simulink model "IEEE9_case"  (R2024b)
settings: Solver=FixedStepAuto  StartTime=0  StopTime=5  FixedStep=1e-7  RelTol=1e-3
values from neighbouring files (symbols this model uses):
  SG_D_1_D = 0.01056    [IEEE9_case_parameters.m]    (also in case1_parameters.m; case2_parameters.m; case3_parameters.m; case4_parameters.m)
  SG_D_1_EnableSaturation = 0    [IEEE9_case_parameters.m]    (also in case1_parameters.m; case2_parameters.m; case3_parameters.m; case4_parameters.m)
  SG_D_1_f0 = 60    [IEEE9_case_parameters.m]    (also in case1_parameters.m; case2_parameters.m; case3_parameters.m; case4_parameters.m)
  SG_D_1_H = 7.5    [IEEE9_case_parameters.m]    (also in case1_parameters.m; case2_parameters.m; case3_parameters.m; case4_parameters.m)
  SG_D_1_K_A = 20    [IEEE9_case_parameters.m]    (also in case1_parameters.m; case2_parameters.m; case3_parameters.m; case4_parameters.m)
  SG_D_1_K_E = 1.000000e+1    (= 10)    [IEEE9_case_parameters.m]    (also in case1_parameters.m; case2_parameters.m; case3_parameters.m; case4_parameters.m)
  SG_D_1_K_F = 2.363    [IEEE9_case_parameters.m]    (also in case1_parameters.m; case2_parameters.m; case3_parameters.m; case4_parameters.m)
  SG_D_1_K_s = 0.5    [IEEE9_case_parameters.m]    (also in case1_parameters.m = 5; case2_parameters.m = 5; case3_parameters.m = 5; case4_parameters.m = 5)
  SG_D_1_R_a = 0.001088    [IEEE9_case_parameters.m]    (also in case1_parameters.m; case2_parameters.m; case3_parameters.m; case4_parameters.m)
  SG_D_1_S_A = 1    [IEEE9_case_parameters.m]    (also in case1_parameters.m; case2_parameters.m; case3_parameters.m; case4_parameters.m)
  SG_D_1_S_B = 0.103    [IEEE9_case_parameters.m]    (also in case1_parameters.m; case2_parameters.m; case3_parameters.m; case4_parameters.m)
  SG_D_1_S_N = 10.659857    [IEEE9_case_parameters.m]    (also in case1_parameters.m; case2_parameters.m; case3_parameters.m; case4_parameters.m)
  SG_D_1_SpeedPara = 200    [IEEE9_case_parameters.m]    (also in case1_parameters.m; case2_parameters.m; case3_parameters.m; case4_parameters.m)
  SG_D_1_T_0 = 0.720173    [IEEE9_case_parameters.m]    (also in case1_parameters.m = 0.755522; case2_parameters.m = 0.808931; case3_parameters.m = 0.869402; case4_parameters.m = 0.729316)
  SG_D_1_T_1 = 0.3    [IEEE9_case_parameters.m]    (also in case1_parameters.m; case2_parameters.m; case3_parameters.m; case4_parameters.m)
  SG_D_1_T_2 = 0.05    [IEEE9_case_parameters.m]    (also in case1_parameters.m; case2_parameters.m; case3_parameters.m; case4_parameters.m)
  SG_D_1_T_3 = 0.02    [IEEE9_case_parameters.m]    (also in case1_parameters.m; case2_parameters.m; case3_parameters.m; case4_parameters.m)
  SG_D_1_T_4 = 0.005    [IEEE9_case_parameters.m]    (also in case1_parameters.m; case2_parameters.m; case3_parameters.m; case4_parameters.m)
  SG_D_1_T_A = 0.02    [IEEE9_case_parameters.m]    (also in case1_parameters.m; case2_parameters.m; case3_parameters.m; case4_parameters.m)
  SG_D_1_T_dd = 8.000000e+0    (= 8)    [IEEE9_case_parameters.m]    (also in case1_parameters.m; case2_parameters.m; case3_parameters.m; case4_parameters.m)
  SG_D_1_T_ddd = 0.04    [IEEE9_case_parameters.m]    (also in case1_parameters.m; case2_parameters.m; case3_parameters.m; case4_parameters.m)
  SG_D_1_T_E = 0.314    [IEEE9_case_parameters.m]    (also in case1_parameters.m; case2_parameters.m; case3_parameters.m; case4_parameters.m)
  SG_D_1_T_F = 0.35    [IEEE9_case_parameters.m]    (also in case1_parameters.m; case2_parameters.m; case3_parameters.m; case4_parameters.m)
  SG_D_1_T_qd = 0.8    [IEEE9_case_parameters.m]    (also in case1_parameters.m; case2_parameters.m; case3_parameters.m; case4_parameters.m)
  SG_D_1_T_qdd = 0.02    [IEEE9_case_parameters.m]    (also in case1_parameters.m; case2_parameters.m; case3_parameters.m; case4_parameters.m)
  SG_D_1_T_speed = 0.1    [IEEE9_case_parameters.m]    (also in case1_parameters.m = 200; case2_parameters.m = 200; case3_parameters.m = 200; case4_parameters.m = 200)
  SG_D_1_T_w = 0.5    [IEEE9_case_parameters.m]    (also in case1_parameters.m; case2_parameters.m; case3_parameters.m; case4_parameters.m)
  SG_D_1_V_ref = 1.990276    [IEEE9_case_parameters.m]    (also in case1_parameters.m = 2.042296; case2_parameters.m = 2.051388; case3_parameters.m = 2.089584; case4_parameters.m = 2.01845)
  SG_D_1_w_ref = 376.991118    [IEEE9_case_parameters.m]    (also in case1_parameters.m; case2_parameters.m; case3_parameters.m; case4_parameters.m)
  SG_D_1_wb = 6.000000e+1    (= 60)    [IEEE9_case_parameters.m]    (also in case1_parameters.m; case2_parameters.m; case3_parameters.m; case4_parameters.m)
  SG_D_1_x_d = 1.9    [IEEE9_case_parameters.m]    (also in case1_parameters.m; case2_parameters.m; case3_parameters.m; case4_parameters.m)
  SG_D_1_x_dd = 0.302    [IEEE9_case_parameters.m]    (also in case1_parameters.m; case2_parameters.m; case3_parameters.m; case4_parameters.m)
  SG_D_1_x_ddd = 0.204    [IEEE9_case_parameters.m]    (also in case1_parameters.m; case2_parameters.m; case3_parameters.m; case4_parameters.m)
  SG_D_1_x_l = 0.05    [IEEE9_case_parameters.m]    (also in case1_parameters.m; case2_parameters.m; case3_parameters.m; case4_parameters.m)
  SG_D_1_x_q = 1.3    [IEEE9_case_parameters.m]    (also in case1_parameters.m; case2_parameters.m; case3_parameters.m; case4_parameters.m)
  SG_D_1_x_qd = 0.5    [IEEE9_case_parameters.m]    (also in case1_parameters.m; case2_parameters.m; case3_parameters.m; case4_parameters.m)
  SG_D_1_x_qdd = 0.3    [IEEE9_case_parameters.m]    (also in case1_parameters.m; case2_parameters.m; case3_parameters.m; case4_parameters.m)
  SG_D_2_D = 0.02    [IEEE9_case_parameters.m]    (also in case1_parameters.m; case2_parameters.m; case3_parameters.m; case4_parameters.m)
  SG_D_2_EnableSaturation = 0    [IEEE9_case_parameters.m]    (also in case1_parameters.m; case2_parameters.m; case3_parameters.m; case4_parameters.m)
  SG_D_2_f0 = 60    [IEEE9_case_parameters.m]    (also in case1_parameters.m; case2_parameters.m; case3_parameters.m; case4_parameters.m)
  SG_D_2_H = 8.000000e+0    (= 8)    [IEEE9_case_parameters.m]    (also in case1_parameters.m; case2_parameters.m; case3_parameters.m; case4_parameters.m)
  SG_D_2_K_A = 20    [IEEE9_case_parameters.m]    (also in case1_parameters.m; case2_parameters.m; case3_parameters.m; case4_parameters.m)
  SG_D_2_K_E = 1.000000e+1    (= 10)    [IEEE9_case_parameters.m]    (also in case1_parameters.m; case2_parameters.m; case3_parameters.m; case4_parameters.m)
  SG_D_2_K_F = 2.363    [IEEE9_case_parameters.m]    (also in case1_parameters.m; case2_parameters.m; case3_parameters.m; case4_parameters.m)
  SG_D_2_K_s = 0.5    [IEEE9_case_parameters.m]    (also in case1_parameters.m = 4; case2_parameters.m = 4; case3_parameters.m = 4; case4_parameters.m = 4)
  SG_D_2_R_a = 0.001088    [IEEE9_case_parameters.m]    (also in case1_parameters.m; case2_parameters.m; case3_parameters.m; case4_parameters.m)
  SG_D_2_S_A = 1    [IEEE9_case_parameters.m]    (also in case1_parameters.m; case2_parameters.m; case3_parameters.m; case4_parameters.m)
  SG_D_2_S_B = 0.103    [IEEE9_case_parameters.m]    (also in case1_parameters.m; case2_parameters.m; case3_parameters.m; case4_parameters.m)
  SG_D_2_S_N = 10.659857    [IEEE9_case_parameters.m]    (also in case1_parameters.m; case2_parameters.m; case3_parameters.m; case4_parameters.m)
  SG_D_2_SpeedPara = 200    [IEEE9_case_parameters.m]    (also in case1_parameters.m; case2_parameters.m; case3_parameters.m; case4_parameters.m)
  SG_D_2_T_0 = 1.632913    [IEEE9_case_parameters.m]    (also in case1_parameters.m = 1.632925; case2_parameters.m = 1.632915; case3_parameters.m = 1.632914; case4_parameters.m = 1.632927)
  SG_D_2_T_1 = 0.2    [IEEE9_case_parameters.m]    (also in case1_parameters.m; case2_parameters.m; case3_parameters.m; case4_parameters.m)
  SG_D_2_T_2 = 0.05    [IEEE9_case_parameters.m]    (also in case1_parameters.m; case2_parameters.m; case3_parameters.m; case4_parameters.m)
  SG_D_2_T_3 = 0.02    [IEEE9_case_parameters.m]    (also in case1_parameters.m; case2_parameters.m; case3_parameters.m; case4_parameters.m)
  SG_D_2_T_4 = 0.005    [IEEE9_case_parameters.m]    (also in case1_parameters.m; case2_parameters.m; case3_parameters.m; case4_parameters.m)
  SG_D_2_T_A = 0.02    [IEEE9_case_parameters.m]    (also in case1_parameters.m; case2_parameters.m; case3_parameters.m; case4_parameters.m)
  SG_D_2_T_dd = 7.9    [IEEE9_case_parameters.m]    (also in case1_parameters.m; case2_parameters.m; case3_parameters.m; case4_parameters.m)
  SG_D_2_T_ddd = 0.04    [IEEE9_case_parameters.m]    (also in case1_parameters.m; case2_parameters.m; case3_parameters.m; case4_parameters.m)
  SG_D_2_T_E = 0.314    [IEEE9_case_parameters.m]    (also in case1_parameters.m; case2_parameters.m; case3_parameters.m; case4_parameters.m)
  SG_D_2_T_F = 0.35    [IEEE9_case_parameters.m]    (also in case1_parameters.m; case2_parameters.m; case3_parameters.m; case4_parameters.m)
  SG_D_2_T_qd = 0.8    [IEEE9_case_parameters.m]    (also in case1_parameters.m; case2_parameters.m; case3_parameters.m; case4_parameters.m)
  SG_D_2_T_qdd = 0.015    [IEEE9_case_parameters.m]    (also in case1_parameters.m; case2_parameters.m; case3_parameters.m; case4_parameters.m)
  SG_D_2_T_speed = 0.1    [IEEE9_case_parameters.m]    (also in case1_parameters.m = 150; case2_parameters.m = 150; case3_parameters.m = 150; case4_parameters.m = 150)
  SG_D_2_T_w = 0.35    [IEEE9_case_parameters.m]    (also in case1_parameters.m; case2_parameters.m; case3_parameters.m; case4_parameters.m)
  SG_D_2_V_ref = 2.58547    [IEEE9_case_parameters.m]    (also in case1_parameters.m = 2.597896; case2_parameters.m = 2.587136; case3_parameters.m = 2.586042; case4_parameters.m = 2.599679)
  SG_D_2_w_ref = 376.991118    [IEEE9_case_parameters.m]    (also in case1_parameters.m; case2_parameters.m; case3_parameters.m; case4_parameters.m)
  SG_D_2_wb = 6.000000e+1    (= 60)    [IEEE9_case_parameters.m]    (also in case1_parameters.m; case2_parameters.m; case3_parameters.m; case4_parameters.m)
  SG_D_2_x_d = 1.8    [IEEE9_case_parameters.m]    (also in case1_parameters.m; case2_parameters.m; case3_parameters.m; case4_parameters.m)
  SG_D_2_x_dd = 0.302    [IEEE9_case_parameters.m]    (also in case1_parameters.m; case2_parameters.m; case3_parameters.m; case4_parameters.m)
  SG_D_2_x_ddd = 0.204    [IEEE9_case_parameters.m]    (also in case1_parameters.m; case2_parameters.m; case3_parameters.m; case4_parameters.m)
  SG_D_2_x_l = 0.05    [IEEE9_case_parameters.m]    (also in case1_parameters.m; case2_parameters.m; case3_parameters.m; case4_parameters.m)
  SG_D_2_x_q = 1.25    [IEEE9_case_parameters.m]    (also in case1_parameters.m; case2_parameters.m; case3_parameters.m; case4_parameters.m)
  SG_D_2_x_qd = 0.5    [IEEE9_case_parameters.m]    (also in case1_parameters.m; case2_parameters.m; case3_parameters.m; case4_parameters.m)
  SG_D_2_x_qdd = 0.3    [IEEE9_case_parameters.m]    (also in case1_parameters.m; case2_parameters.m; case3_parameters.m; case4_parameters.m)
  SG_D_3_D = 0.02    [IEEE9_case_parameters.m]    (also in case1_parameters.m; case2_parameters.m; case3_parameters.m; case4_parameters.m)
  SG_D_3_EnableSaturation = 0    [IEEE9_case_parameters.m]    (also in case1_parameters.m; case2_parameters.m; case3_parameters.m; case4_parameters.m)
  SG_D_3_f0 = 60    [IEEE9_case_parameters.m]    (also in case1_parameters.m; case2_parameters.m; case3_parameters.m; case4_parameters.m)
  SG_D_3_H = 7.7    [IEEE9_case_parameters.m]    (also in case1_parameters.m; case2_parameters.m; case3_parameters.m; case4_parameters.m)
  SG_D_3_K_A = 20    [IEEE9_case_parameters.m]    (also in case1_parameters.m; case2_parameters.m; case3_parameters.m; case4_parameters.m)
  SG_D_3_K_E = 1.000000e+1    (= 10)    [IEEE9_case_parameters.m]    (also in case1_parameters.m; case2_parameters.m; case3_parameters.m; case4_parameters.m)
  SG_D_3_K_F = 2.363    [IEEE9_case_parameters.m]    (also in case1_parameters.m; case2_parameters.m; case3_parameters.m; case4_parameters.m)
  SG_D_3_K_s = 0.2    [IEEE9_case_parameters.m]    (also in case1_parameters.m = 2; case2_parameters.m = 2; case3_parameters.m = 2; case4_parameters.m = 2)
  SG_D_3_R_a = 0.001088    [IEEE9_case_parameters.m]    (also in case1_parameters.m; case2_parameters.m; case3_parameters.m; case4_parameters.m)
  SG_D_3_S_A = 1    [IEEE9_case_parameters.m]    (also in case1_parameters.m; case2_parameters.m; case3_parameters.m; case4_parameters.m)
  SG_D_3_S_B = 0.103    [IEEE9_case_parameters.m]    (also in case1_parameters.m; case2_parameters.m; case3_parameters.m; case4_parameters.m)
  SG_D_3_S_N = 10.659857    [IEEE9_case_parameters.m]    (also in case1_parameters.m; case2_parameters.m; case3_parameters.m; case4_parameters.m)
  SG_D_3_SpeedPara = 200    [IEEE9_case_parameters.m]    (also in case1_parameters.m; case2_parameters.m; case3_parameters.m; case4_parameters.m)
  SG_D_3_T_0 = 0.850788    [IEEE9_case_parameters.m]    (also in case1_parameters.m = 0.850786; case2_parameters.m = 0.850787; case3_parameters.m; case4_parameters.m = 0.850786)
  SG_D_3_T_1 = 0.2    [IEEE9_case_parameters.m]    (also in case1_parameters.m; case2_parameters.m; case3_parameters.m; case4_parameters.m)
  SG_D_3_T_2 = 0.05    [IEEE9_case_parameters.m]    (also in case1_parameters.m; case2_parameters.m; case3_parameters.m; case4_parameters.m)
  SG_D_3_T_3 = 0.02    [IEEE9_case_parameters.m]    (also in case1_parameters.m; case2_parameters.m; case3_parameters.m; case4_parameters.m)
  SG_D_3_T_4 = 0.005    [IEEE9_case_parameters.m]    (also in case1_parameters.m; case2_parameters.m; case3_parameters.m; case4_parameters.m)
  SG_D_3_T_A = 0.02    [IEEE9_case_parameters.m]    (also in case1_parameters.m; case2_parameters.m; case3_parameters.m; case4_parameters.m)
  SG_D_3_T_dd = 8.1    [IEEE9_case_parameters.m]    (also in case1_parameters.m; case2_parameters.m; case3_parameters.m; case4_parameters.m)
  SG_D_3_T_ddd = 0.04    [IEEE9_case_parameters.m]    (also in case1_parameters.m; case2_parameters.m; case3_parameters.m; case4_parameters.m)
  SG_D_3_T_E = 0.314    [IEEE9_case_parameters.m]    (also in case1_parameters.m; case2_parameters.m; case3_parameters.m; case4_parameters.m)
  SG_D_3_T_F = 0.35    [IEEE9_case_parameters.m]    (also in case1_parameters.m; case2_parameters.m; case3_parameters.m; case4_parameters.m)
  SG_D_3_T_qd = 0.8    [IEEE9_case_parameters.m]    (also in case1_parameters.m; case2_parameters.m; case3_parameters.m; case4_parameters.m)
  SG_D_3_T_qdd = 0.015    [IEEE9_case_parameters.m]    (also in case1_parameters.m; case2_parameters.m; case3_parameters.m; case4_parameters.m)
  SG_D_3_T_speed = 0.1    [IEEE9_case_parameters.m]    (also in case1_parameters.m = 180; case2_parameters.m = 180; case3_parameters.m = 180; case4_parameters.m = 180)
  SG_D_3_T_w = 0.4    [IEEE9_case_parameters.m]    (also in case1_parameters.m; case2_parameters.m; case3_parameters.m; case4_parameters.m)
  SG_D_3_V_ref = 1.892727    [IEEE9_case_parameters.m]    (also in case1_parameters.m = 1.906439; case2_parameters.m = 1.895535; case3_parameters.m = 1.892105; case4_parameters.m = 1.906598)
  SG_D_3_w_ref = 376.991118    [IEEE9_case_parameters.m]    (also in case1_parameters.m; case2_parameters.m; case3_parameters.m; case4_parameters.m)
  SG_D_3_wb = 6.000000e+1    (= 60)    [IEEE9_case_parameters.m]    (also in case1_parameters.m; case2_parameters.m; case3_parameters.m; case4_parameters.m)
  SG_D_3_x_d = 1.85    [IEEE9_case_parameters.m]    (also in case1_parameters.m; case2_parameters.m; case3_parameters.m; case4_parameters.m)
  SG_D_3_x_dd = 0.302    [IEEE9_case_parameters.m]    (also in case1_parameters.m; case2_parameters.m; case3_parameters.m; case4_parameters.m)
  SG_D_3_x_ddd = 0.204    [IEEE9_case_parameters.m]    (also in case1_parameters.m; case2_parameters.m; case3_parameters.m; case4_parameters.m)
  SG_D_3_x_l = 0.05    [IEEE9_case_parameters.m]    (also in case1_parameters.m; case2_parameters.m; case3_parameters.m; case4_parameters.m)
  SG_D_3_x_q = 1.2    [IEEE9_case_parameters.m]    (also in case1_parameters.m; case2_parameters.m; case3_parameters.m; case4_parameters.m)
  SG_D_3_x_qd = 0.5    [IEEE9_case_parameters.m]    (also in case1_parameters.m; case2_parameters.m; case3_parameters.m; case4_parameters.m)
  SG_D_3_x_qdd = 0.3    [IEEE9_case_parameters.m]    (also in case1_parameters.m; case2_parameters.m; case3_parameters.m; case4_parameters.m)
(part 8 of 12)

== system IEEE9_case/SG_D_2/d_psi_1d_SG_D_2_block ==
  note: d_psi_1d_SG_D_2 in IEEE9_case
      | $-\frac{\psi _{\mathrm{1d},\mathrm{SG},D,2}-\psi _{\mathrm{fd},\mathrm{SG},D,2}+\frac{\left(x_{\mathrm{dd}}-x_{l}\right)\,\left(\frac{\psi _{\mathrm{1d},\mathrm{SG},D,2}\,\left(x_{\mathrm{dd}}-x_{\mathrm{ddd}}\right)}{x_{\mathrm{dd}}-x_{l}}-\psi _{d,\mathrm{SG},D,2}+\frac{\psi _{\mathrm{fd},\mathrm{SG},D,2}\,\left(x_{\mathrm{ddd}}-x_{l}\right)}{x_{\mathrm{dd}}-x_{l}}\right)}{x_{\mathrm{ddd}}}}{T_{\mathrm{ddd}}}$
      | Automatically generated on 2025-11-01 08:48:44 .
  State_psi_1d_SG_D_2_41588 : Inport
  State_psi_fd_SG_D_2_683d9 : Inport  Port=2
  State_psi_1d_SG_D_2_bbec1 : Inport  Port=3
  State_psi_d_SG_D_2_88e69 : Inport  Port=4
  State_psi_fd_SG_D_2_1a1ec : Inport  Port=5
  Add_96336 : Sum
  Add_f9459 : Sum
  Add_fbbb9 : Sum
  Constant_-1_93479 : Constant  Value=-1
  Constant_-1_ecd3b : Constant  Value=-1
  Constant_T_ddd_afdda : Constant  Value=T_ddd
  Constant_x_dd_10c30 : Constant  Value=x_dd
  Constant_x_dd_4707f : Constant  Value=x_dd
  Constant_x_dd_892b1 : Constant  Value=x_dd
  Constant_x_dd_8c4fd : Constant  Value=x_dd
  Constant_x_ddd_37c6d : Constant  Value=x_ddd
  Constant_x_ddd_41833 : Constant  Value=x_ddd
  Constant_x_ddd_cac59 : Constant  Value=x_ddd
  Constant_x_l_23a16 : Constant  Value=x_l
  Constant_x_l_319dd : Constant  Value=x_l
  Constant_x_l_3d5de : Constant  Value=x_l
  Constant_x_l_5cdf5 : Constant  Value=x_l
  Divide_03784 : Product  Inputs=*/
  Divide_3e18e : Product  Inputs=*/
  Divide_57b11 : Product  Inputs=*/
  Divide_7da2c : Product  Inputs=*/
  Product_037dc : Product
  Product_06fd5 : Product
  Product_25ddc : Product
  Product_4ec97 : Product
  Product_7d4ba : Product
  Subtract_08c94 : Sum  Inputs=+-
  Subtract_30855 : Sum  Inputs=+-
  Subtract_32cab : Sum  Inputs=+-
  Subtract_369e1 : Sum  Inputs=+-
  Subtract_819dd : Sum  Inputs=+-
  Subtract_e1548 : Sum  Inputs=+-
  Blockout_d_psi_1d_SG_D_2_e4c33 : Outport
  wires:
  Subtract_819dd/1 -> Product_06fd5/2
  Constant_x_l_5cdf5/1 -> Subtract_08c94/2
  Divide_3e18e/1 -> Add_96336/2
  Subtract_e1548/1 -> Product_4ec97/2
  Constant_-1_ecd3b/1 -> Product_037dc/1
  Constant_x_dd_10c30/1 -> Subtract_369e1/1
  Divide_57b11/1 -> Blockout_d_psi_1d_SG_D_2_e4c33/1
  State_psi_fd_SG_D_2_683d9/1 -> Add_fbbb9/2
  State_psi_1d_SG_D_2_bbec1/1 -> Product_037dc/2
  Divide_03784/1 -> Subtract_e1548/2
  Constant_x_ddd_37c6d/1 -> Subtract_369e1/2
  State_psi_1d_SG_D_2_41588/1 -> Product_7d4ba/2
  Product_037dc/1 -> Product_25ddc/1
  Subtract_369e1/1 -> Product_25ddc/2
  Constant_x_dd_892b1/1 -> Subtract_08c94/1
  Constant_x_ddd_41833/1 -> Subtract_819dd/1
  Constant_x_l_23a16/1 -> Subtract_819dd/2
  Product_25ddc/1 -> Divide_7da2c/1
  Subtract_08c94/1 -> Divide_7da2c/2
  State_psi_fd_SG_D_2_1a1ec/1 -> Product_06fd5/1
  Constant_x_dd_8c4fd/1 -> Subtract_30855/1
  Constant_x_l_319dd/1 -> Subtract_32cab/2
  Constant_x_l_3d5de/1 -> Subtract_30855/2
  Constant_x_ddd_cac59/1 -> Divide_3e18e/2
  Divide_7da2c/1 -> Add_f9459/1
  State_psi_d_SG_D_2_88e69/1 -> Add_f9459/2
  Product_06fd5/1 -> Divide_03784/1
  Subtract_30855/1 -> Divide_03784/2
  Constant_x_dd_4707f/1 -> Subtract_32cab/1
  Add_f9459/1 -> Subtract_e1548/1
  Constant_-1_93479/1 -> Product_7d4ba/1
  Subtract_32cab/1 -> Product_4ec97/1
  Product_7d4ba/1 -> Add_fbbb9/1
  Product_4ec97/1 -> Divide_3e18e/1
  Add_fbbb9/1 -> Add_96336/1
  Add_96336/1 -> Divide_57b11/1
  Constant_T_ddd_afdda/1 -> Divide_57b11/2

== system IEEE9_case/SG_D_2/d_psi_d_SG_D_2_block ==
  note: d_psi_d_SG_D_2 in IEEE9_case
      | $2\,\pi \,f_{0}\,\left(v_{d,\mathrm{SG},D,2}\,\sin\left(\theta _{\mathrm{SG},D,2}\right)-v_{q,\mathrm{SG},D,2}\,\cos\left(\theta _{\mathrm{SG},D,2}\right)+\frac{R_{a}\,\left(\frac{\psi _{\mathrm{1d},\mathrm{SG},D,2}\,\left(x_{\mathrm{dd}}-x_{\mathrm{ddd}}\right)}{x_{\mathrm{dd}}-x_{l}}-\psi _{d,\mathrm{SG},D,2}+\frac{\psi _{\mathrm{fd},\mathrm{SG},D,2}\,\left(x_{\mathrm{ddd}}-x_{l}\right)}{x_{\mathrm{dd}}-x_{l}}\right)}{x_{\mathrm{ddd}}}+\frac{\psi _{q,\mathrm{SG},D,2}\,w_{\mathrm{SG},D,2}}{2\,f_{0}\,\pi }\right)$
      | Automatically generated on 2025-11-01 08:48:33 .
  State_psi_1d_SG_D_2_9e75a : Inport
  State_psi_d_SG_D_2_1509d : Inport  Port=2
  State_psi_fd_SG_D_2_6b3f8 : Inport  Port=3
  Input_v_d_SG_D_2_43371 : Inport  Port=4
  State_theta_SG_D_2_d1f6e : Inport  Port=5
  Input_v_q_SG_D_2_68fd3 : Inport  Port=6
  State_theta_SG_D_2_8a255 : Inport  Port=7
  State_psi_q_SG_D_2_03603 : Inport  Port=8
  State_w_SG_D_2_4590a : Inport  Port=9
  Add_2da11 : Sum
  Add_2facd : Sum
  Constant_-1_5cc25 : Constant  Value=-1
  Constant_-2.0_76f71 : Constant  Value=-2.0
  Constant_2.0_2c16b : Constant  Value=2.0
  Constant_R_a_80df7 : Constant  Value=R_a
  Constant_f0_14fbf : Constant  Value=f0
  Constant_f0_1f62f : Constant  Value=f0
  Constant_pi_4d850 : Constant  Value=pi
  Constant_pi_a77f8 : Constant  Value=pi
  Constant_x_dd_184ae : Constant  Value=x_dd
  Constant_x_dd_457a1 : Constant  Value=x_dd
  Constant_x_dd_fefd6 : Constant  Value=x_dd
  Constant_x_ddd_22c81 : Constant  Value=x_ddd
  Constant_x_ddd_357e5 : Constant  Value=x_ddd
  Constant_x_ddd_9abf6 : Constant  Value=x_ddd
  Constant_x_l_07a6a : Constant  Value=x_l
  Constant_x_l_98279 : Constant  Value=x_l
  Constant_x_l_f8c6f : Constant  Value=x_l
  Divide_7a585 : Product  Inputs=*/
  Divide_804c4 : Product  Inputs=*/
  Divide_989cf : Product  Inputs=*/
  Divide_9e0dc : Product  Inputs=*/
  MathFunc_cos_bdfb6 : Trigonometry  Operator=cos
  MathFunc_sin_2ba6d : Trigonometry
  Product_16a86 : Product
  Product_37c68 : Product
  Product_3ed6d : Product
  Product_48c1e : Product
  Product_52104 : Product
  Product_61df5 : Product
  Product_99f53 : Product
  Product_a3b7f : Product
  Product_d99c5 : Product
  Product_eacdf : Product
  Product_eb5c0 : Product
  Product_f284e : Product
  Subtract_28354 : Sum  Inputs=+-
  Subtract_2d0de : Sum  Inputs=+-
  Subtract_31ac1 : Sum  Inputs=+-
  Subtract_4cf5e : Sum  Inputs=+-
  Subtract_ca281 : Sum  Inputs=+-
  Subtract_dcedb : Sum  Inputs=+-
  Subtract_f88cf : Sum  Inputs=+-
  Blockout_d_psi_d_SG_D_2_65f41 : Outport
  wires:
  MathFunc_sin_2ba6d/1 -> Product_48c1e/2
  Constant_x_dd_fefd6/1 -> Subtract_4cf5e/1
  Constant_-1_5cc25/1 -> Product_52104/1
  Constant_x_l_f8c6f/1 -> Subtract_4cf5e/2
  State_psi_1d_SG_D_2_9e75a/1 -> Product_52104/2
  Constant_f0_1f62f/1 -> Product_a3b7f/2
  Constant_2.0_2c16b/1 -> Product_f284e/1
  Constant_x_l_07a6a/1 -> Subtract_ca281/2
  Constant_x_dd_457a1/1 -> Subtract_f88cf/1
  Product_eacdf/1 -> Blockout_d_psi_d_SG_D_2_65f41/1
  Constant_pi_4d850/1 -> Product_f284e/2
  Constant_x_ddd_357e5/1 -> Subtract_f88cf/2
  Subtract_28354/1 -> Product_eacdf/2
  Product_52104/1 -> Product_37c68/1
  Product_f284e/1 -> Product_16a86/1
  Subtract_f88cf/1 -> Product_37c68/2
  Divide_7a585/1 -> Subtract_28354/2
  Constant_x_ddd_9abf6/1 -> Subtract_31ac1/1
  Constant_x_l_98279/1 -> Subtract_31ac1/2
  Product_37c68/1 -> Divide_804c4/1
  Subtract_dcedb/1 -> Add_2da11/1
  Subtract_4cf5e/1 -> Divide_804c4/2
  State_psi_fd_SG_D_2_6b3f8/1 -> Product_d99c5/1
  Subtract_31ac1/1 -> Product_d99c5/2
  Constant_x_dd_184ae/1 -> Subtract_ca281/1
  Divide_804c4/1 -> Add_2facd/1
  State_psi_d_SG_D_2_1509d/1 -> Add_2facd/2
  Product_d99c5/1 -> Divide_989cf/1
  Subtract_ca281/1 -> Divide_989cf/2
  Add_2facd/1 -> Subtract_2d0de/1
  Divide_989cf/1 -> Subtract_2d0de/2
  Constant_R_a_80df7/1 -> Product_61df5/1
  Subtract_2d0de/1 -> Product_61df5/2
  Divide_9e0dc/1 -> Subtract_dcedb/1
  State_theta_SG_D_2_d1f6e/1 -> MathFunc_sin_2ba6d/1
  Product_61df5/1 -> Divide_9e0dc/1
  Constant_-2.0_76f71/1 -> Product_3ed6d/1
  Input_v_d_SG_D_2_43371/1 -> Product_48c1e/1
  Constant_x_ddd_22c81/1 -> Divide_9e0dc/2
  State_theta_SG_D_2_8a255/1 -> MathFunc_cos_bdfb6/1
  Product_a3b7f/1 -> Product_eacdf/1
  Product_48c1e/1 -> Subtract_dcedb/2
  Product_3ed6d/1 -> Product_a3b7f/1
  Input_v_q_SG_D_2_68fd3/1 -> Product_eb5c0/1
  MathFunc_cos_bdfb6/1 -> Product_eb5c0/2
  State_psi_q_SG_D_2_03603/1 -> Product_99f53/1
  State_w_SG_D_2_4590a/1 -> Product_99f53/2
  Constant_f0_14fbf/1 -> Product_16a86/2
  Constant_pi_a77f8/1 -> Product_3ed6d/2
  Product_eb5c0/1 -> Add_2da11/2
  Product_99f53/1 -> Divide_7a585/1
  Product_16a86/1 -> Divide_7a585/2
  Add_2da11/1 -> Subtract_28354/1

== system IEEE9_case/SG_D_2/d_psi_fd_SG_D_2_block ==
  note: d_psi_fd_SG_D_2 in IEEE9_case
      | $-\frac{\psi _{\mathrm{fd},\mathrm{SG},D,2}-E_{\mathrm{fd},\mathrm{SG},D,2}+\left(x_{d}-x_{\mathrm{dd}}\right)\,\left(\frac{\frac{\psi _{\mathrm{1d},\mathrm{SG},D,2}\,\left(x_{\mathrm{dd}}-x_{\mathrm{ddd}}\right)}{x_{\mathrm{dd}}-x_{l}}-\psi _{d,\mathrm{SG},D,2}+\frac{\psi _{\mathrm{fd},\mathrm{SG},D,2}\,\left(x_{\mathrm{ddd}}-x_{l}\right)}{x_{\mathrm{dd}}-x_{l}}}{x_{\mathrm{ddd}}}-\frac{\left(x_{\mathrm{dd}}-x_{\mathrm{ddd}}\right)\,\left(\psi _{\mathrm{1d},\mathrm{SG},D,2}-\psi _{\mathrm{fd},\mathrm{SG},D,2}+\frac{\left(x_{\mathrm{dd}}-x_{l}\right)\,\left(\frac{\psi _{\mathrm{1d},\mathrm{SG},D,2}\,\left(x_{\mathrm{dd}}-x_{\mathrm{ddd}}\right)}{x_{\mathrm{dd}}-x_{l}}-\psi _{d,\mathrm{SG},D,2}+\frac{\psi _{\mathrm{fd},\mathrm{SG},D,2}\,\left(x_{\mathrm{ddd}}-x_{l}\right)}{x_{\mathrm{dd}}-x_{l}}\right)}{x_{\mathrm{ddd}}}\right)}{{\left(x_{\mathrm{dd}}-x_{l}\right)}^2}\right)}{T_{\mathrm{dd}}}$
      | Automatically generated on 2025-11-01 08:48:41 .
  State_E_fd_SG_D_2_7c2d9 : Inport
  State_psi_fd_SG_D_2_96da5 : Inport  Port=2
  State_psi_1d_SG_D_2_c35a5 : Inport  Port=3
  State_psi_fd_SG_D_2_18c77 : Inport  Port=4
  State_psi_1d_SG_D_2_e2991 : Inport  Port=5
  State_psi_d_SG_D_2_08540 : Inport  Port=6
  State_psi_fd_SG_D_2_4a3c7 : Inport  Port=7
  State_psi_1d_SG_D_2_7e692 : Inport  Port=8
  State_psi_d_SG_D_2_798aa : Inport  Port=9
  State_psi_fd_SG_D_2_7bfa6 : Inport  Port=10
  Add_3437b : Sum
  Add_b4710 : Sum
  Constant_-1_3da81 : Constant  Value=-1
  Constant_-1_be5a6 : Constant  Value=-1
  Constant_-1_bea49 : Constant  Value=-1
  Constant_2.0_01584 : Constant  Value=2.0
  Constant_T_dd_d035e : Constant  Value=T_dd
  Constant_x_d_0d8bb : Constant  Value=x_d
  Constant_x_dd_05a6e : Constant  Value=x_dd
  Constant_x_dd_1cf4b : Constant  Value=x_dd
  Constant_x_dd_2cbbb : Constant  Value=x_dd
  Constant_x_dd_6c0d2 : Constant  Value=x_dd
  Constant_x_dd_7dfe9 : Constant  Value=x_dd
  Constant_x_dd_a591e : Constant  Value=x_dd
  Constant_x_dd_a8140 : Constant  Value=x_dd
  Constant_x_dd_ad2fc : Constant  Value=x_dd
  Constant_x_dd_eb5f5 : Constant  Value=x_dd
  Constant_x_dd_fb12a : Constant  Value=x_dd
  Constant_x_ddd_19c49 : Constant  Value=x_ddd
  Constant_x_ddd_4a21d : Constant  Value=x_ddd
  Constant_x_ddd_7f605 : Constant  Value=x_ddd
  Constant_x_ddd_d4a12 : Constant  Value=x_ddd
  Constant_x_ddd_db765 : Constant  Value=x_ddd
  Constant_x_ddd_fba81 : Constant  Value=x_ddd
  Constant_x_ddd_fc137 : Constant  Value=x_ddd
  Constant_x_l_14819 : Constant  Value=x_l
  Constant_x_l_23627 : Constant  Value=x_l
  Constant_x_l_3a088 : Constant  Value=x_l
  Constant_x_l_3b6d7 : Constant  Value=x_l
  Constant_x_l_5fa99 : Constant  Value=x_l
  Constant_x_l_7ff39 : Constant  Value=x_l
  Constant_x_l_ab82a : Constant  Value=x_l
  Constant_x_l_b1209 : Constant  Value=x_l
  Divide_27aac : Product  Inputs=*/
  Divide_6640d : Product  Inputs=*/
  Divide_699e9 : Product  Inputs=*/
  Divide_790c7 : Product  Inputs=*/
  Divide_98f6e : Product  Inputs=*/
  Divide_ca46e : Product  Inputs=*/
  Divide_d0a5e : Product  Inputs=*/
  Divide_ec689 : Product  Inputs=*/
  Power_9796c : Math  Operator=pow
  Product_0680b : Product
  Product_124b3 : Product
  Product_1d653 : Product
  Product_56d6a : Product
  Product_58f38 : Product
  Product_5ca66 : Product
  Product_98ca8 : Product
  Product_a117f : Product
  Product_cd2b2 : Product
  Product_de4b2 : Product
  Subtract_001d7 : Sum  Inputs=+-
  Subtract_1e62f : Sum  Inputs=+-
  Subtract_259e2 : Sum  Inputs=+-
  Subtract_37e25 : Sum  Inputs=+-
  Subtract_3a2fb : Sum  Inputs=+-
  Subtract_5059b : Sum  Inputs=+-
  Subtract_51e1e : Sum  Inputs=+-
  Subtract_544fa : Sum  Inputs=+-
  Subtract_5c96f : Sum  Inputs=+-
  Subtract_66718 : Sum  Inputs=+-
  Subtract_b0994 : Sum  Inputs=+-
  Subtract_c7482 : Sum  Inputs=+-
  Subtract_cc977 : Sum  Inputs=+-
  Subtract_d985e : Sum  Inputs=+-
  Subtract_e3d78 : Sum  Inputs=+-
  Subtract_e98e8 : Sum  Inputs=+-
  Subtract_eb1d0 : Sum  Inputs=+-
  Subtract_ed9f4 : Sum  Inputs=+-
  Subtract_fb940 : Sum  Inputs=+-
  Blockout_d_psi_fd_SG_D_2_fb63c : Outport
  wires:
  Constant_x_dd_a8140/1 -> Subtract_ed9f4/1
  Constant_-1_3da81/1 -> Product_0680b/1
  Constant_x_l_b1209/1 -> Subtract_b0994/2
  Divide_699e9/1 -> Add_b4710/1
  Subtract_1e62f/1 -> Product_a117f/2
  Constant_x_l_7ff39/1 -> Subtract_ed9f4/2
  Product_a117f/1 -> Divide_98f6e/1
  State_psi_1d_SG_D_2_e2991/1 -> Product_0680b/2
  Constant_x_dd_ad2fc/1 -> Subtract_fb940/1
  Product_98ca8/1 -> Divide_699e9/1
  Constant_x_dd_1cf4b/1 -> Subtract_cc977/1
  Constant_x_ddd_4a21d/1 -> Subtract_fb940/2
  Constant_x_dd_a591e/1 -> Subtract_37e25/1
  Product_0680b/1 -> Product_58f38/1
  Subtract_fb940/1 -> Product_58f38/2
  State_psi_d_SG_D_2_798aa/1 -> Add_b4710/2
  Constant_x_ddd_7f605/1 -> Subtract_1e62f/1
  Constant_x_l_5fa99/1 -> Subtract_1e62f/2
  Product_58f38/1 -> Divide_790c7/1
  Subtract_ed9f4/1 -> Divide_790c7/2
  State_psi_fd_SG_D_2_4a3c7/1 -> Product_a117f/1
  Subtract_51e1e/1 -> Product_1d653/2
  Constant_x_dd_05a6e/1 -> Subtract_66718/1
  Constant_x_l_3b6d7/1 -> Subtract_66718/2
  Product_56d6a/1 -> Product_1d653/1
  Divide_790c7/1 -> Add_3437b/1
  State_psi_d_SG_D_2_08540/1 -> Add_3437b/2
  Subtract_66718/1 -> Divide_98f6e/2
  Constant_x_dd_fb12a/1 -> Subtract_b0994/1
  Constant_x_ddd_d4a12/1 -> Subtract_259e2/1
  Add_3437b/1 -> Subtract_eb1d0/1
  Divide_98f6e/1 -> Subtract_eb1d0/2
  Constant_-1_be5a6/1 -> Product_5ca66/1
  Product_cd2b2/1 -> Divide_ec689/1
  State_psi_1d_SG_D_2_7e692/1 -> Product_5ca66/2
  Subtract_cc977/1 -> Product_56d6a/2
  Constant_x_dd_2cbbb/1 -> Subtract_5c96f/1
  Divide_ec689/1 -> Subtract_3a2fb/2
  Constant_-1_bea49/1 -> Product_56d6a/1
  Constant_x_ddd_db765/1 -> Subtract_5c96f/2
  Constant_x_ddd_fba81/1 -> Divide_ca46e/2
  Subtract_b0994/1 -> Product_de4b2/1
  Subtract_eb1d0/1 -> Product_de4b2/2
  State_psi_fd_SG_D_2_18c77/1 -> Subtract_e98e8/2
  Product_5ca66/1 -> Product_98ca8/1
  Subtract_5c96f/1 -> Product_98ca8/2
  Constant_2.0_01584/1 -> Power_9796c/2
  State_psi_1d_SG_D_2_c35a5/1 -> Subtract_e98e8/1
  Constant_x_dd_eb5f5/1 -> Subtract_5059b/1
  Subtract_259e2/1 -> Product_cd2b2/2
  Constant_x_l_14819/1 -> Subtract_5059b/2
  Constant_x_l_23627/1 -> Subtract_259e2/2
  Constant_x_ddd_fc137/1 -> Subtract_cc977/2
  Subtract_37e25/1 -> Divide_ec689/2
  Product_de4b2/1 -> Divide_ca46e/1
  Subtract_5059b/1 -> Divide_699e9/2
  State_psi_fd_SG_D_2_7bfa6/1 -> Product_cd2b2/1
  Constant_x_l_3a088/1 -> Subtract_37e25/2
  Constant_x_dd_6c0d2/1 -> Subtract_544fa/1
  Subtract_e98e8/1 -> Subtract_51e1e/1
  Divide_ca46e/1 -> Subtract_51e1e/2
  Constant_x_l_ab82a/1 -> Subtract_544fa/2
  Subtract_544fa/1 -> Power_9796c/1
  Add_b4710/1 -> Subtract_3a2fb/1
  Product_1d653/1 -> Divide_6640d/1
  Power_9796c/1 -> Divide_6640d/2
  Subtract_3a2fb/1 -> Divide_d0a5e/1
  Constant_x_ddd_19c49/1 -> Divide_d0a5e/2
  Constant_x_d_0d8bb/1 -> Subtract_c7482/1
  Constant_x_dd_7dfe9/1 -> Subtract_c7482/2
  Divide_6640d/1 -> Subtract_001d7/1
  Divide_d0a5e/1 -> Subtract_001d7/2
  State_E_fd_SG_D_2_7c2d9/1 -> Subtract_e3d78/1
  State_psi_fd_SG_D_2_96da5/1 -> Subtract_e3d78/2
  Subtract_c7482/1 -> Product_124b3/1
  Subtract_001d7/1 -> Product_124b3/2
  Subtract_e3d78/1 -> Subtract_d985e/1
  Product_124b3/1 -> Subtract_d985e/2
  Subtract_d985e/1 -> Divide_27aac/1
  Constant_T_dd_d035e/1 -> Divide_27aac/2
  Divide_27aac/1 -> Blockout_d_psi_fd_SG_D_2_fb63c/1

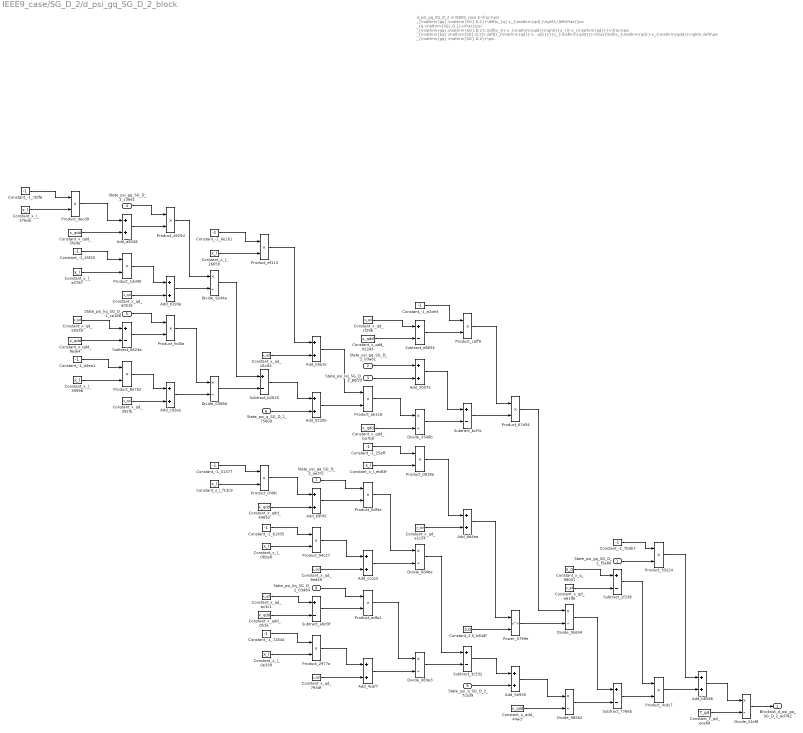
== system IEEE9_case/SG_D_2/d_psi_gq_SG_D_2_block ==
  note: d_psi_gq_SG_D_2 in IEEE9_case
      | $-\frac{\psi _{\mathrm{gq},\mathrm{SG},D,2}+\left(x_{q}-x_{\mathrm{qd}}\right)\,\left(\frac{\psi _{q,\mathrm{SG},D,2}+\frac{\psi _{\mathrm{gq},\mathrm{SG},D,2}\,\left(x_{l}-x_{\mathrm{qdd}}\right)}{x_{l}-x_{\mathrm{qd}}}+\frac{\psi _{\mathrm{kq},\mathrm{SG},D,2}\,\left(x_{\mathrm{qd}}-x_{\mathrm{qdd}}\right)}{x_{l}-x_{\mathrm{qd}}}}{x_{\mathrm{qdd}}}+\frac{\left(x_{\mathrm{qd}}-x_{\mathrm{qdd}}\right)\,\left(\psi _{\mathrm{gq},\mathrm{SG},D,2}+\psi _{\mathrm{kq},\mathrm{SG},D,2}+\frac{\left(x_{l}-x_{\mathrm{qd}}\right)\,\left(\psi _{q,\mathrm{SG},D,2}+\frac{\psi _{\mathrm{gq},\mathrm{SG},D,2}\,\left(x_{l}-x_{\mathrm{qdd}}\right)}{x_{l}-x_{\mathrm{qd}}}+\frac{\psi _{\mathrm{kq},\mathrm{SG},D,2}\,\left(x_{\mathrm{qd}}-x_{\mathrm{qdd}}\right)}{x_{l}-x_{\mathrm{qd}}}\right)}{x_{\mathrm{qdd}}}\right)}{{\left(x_{l}-x_{\mathrm{qd}}\right)}^2}\right)}{T_{\mathrm{qd}}}$
      | Automatically generated on 2025-11-01 08:48:50 .
  State_psi_gq_SG_D_2_f5a80 : Inport
  State_psi_gq_SG_D_2_b3a61 : Inport  Port=2
  State_psi_kq_SG_D_2_80cf3 : Inport  Port=3
  State_psi_gq_SG_D_2_c36e1 : Inport  Port=4
  State_psi_kq_SG_D_2_ca188 : Inport  Port=5
  State_psi_q_SG_D_2_75609 : Inport  Port=6
  State_psi_gq_SG_D_2_ee37c : Inport  Port=7
  State_psi_kq_SG_D_2_03d84 : Inport  Port=8
  State_psi_q_SG_D_2_7ca39 : Inport  Port=9
  Add_0193e : Sum
  Add_0220b : Sum
  Add_20575 : Sum
  Add_4caf7 : Sum
  Add_5e930 : Sum
  Add_6d4ea : Sum
  Add_a8348 : Sum
  Add_b5b3c : Sum
  Add_b6586 : Sum
  Add_b9f45 : Sum
  Add_c92ee : Sum
  Add_ccca3 : Sum
  Constant_-1_01377 : Constant  Value=-1
  Constant_-1_25aff : Constant  Value=-1
  Constant_-1_45f20 : Constant  Value=-1
  Constant_-1_6e161 : Constant  Value=-1
  Constant_-1_72844 : Constant  Value=-1
  Constant_-1_7bdb7 : Constant  Value=-1
  Constant_-1_7bff6 : Constant  Value=-1
  Constant_-1_b1935 : Constant  Value=-1
  Constant_-1_d4ea1 : Constant  Value=-1
  Constant_-1_e2de3 : Constant  Value=-1
  Constant_2.0_b84df : Constant  Value=2.0
  Constant_T_qd_eceb8 : Constant  Value=T_qd
  Constant_x_l_082e8 : Constant  Value=x_l
  Constant_x_l_0e339 : Constant  Value=x_l
  Constant_x_l_16659 : Constant  Value=x_l
  Constant_x_l_376da : Constant  Value=x_l
  Constant_x_l_39996 : Constant  Value=x_l
  Constant_x_l_e3787 : Constant  Value=x_l
  Constant_x_l_eb83f : Constant  Value=x_l
  Constant_x_l_f13c9 : Constant  Value=x_l
  Constant_x_q_98001 : Constant  Value=x_q
  Constant_x_qd_391fb : Constant  Value=x_qd
  Constant_x_qd_50550 : Constant  Value=x_qd
  Constant_x_qd_793df : Constant  Value=x_qd
  Constant_x_qd_9ed49 : Constant  Value=x_qd
  Constant_x_qd_a0516 : Constant  Value=x_qd
  Constant_x_qd_ac3c1 : Constant  Value=x_qd
  Constant_x_qd_cf296 : Constant  Value=x_qd
  Constant_x_qd_d1c64 : Constant  Value=x_qd
  Constant_x_qd_e1c54 : Constant  Value=x_qd
  Constant_x_qd_e6196 : Constant  Value=x_qd
  Constant_x_qdd_0fcfe : Constant  Value=x_qdd
  Constant_x_qdd_40652 : Constant  Value=x_qdd
  Constant_x_qdd_44acf : Constant  Value=x_qdd
  Constant_x_qdd_5fede : Constant  Value=x_qdd
  Constant_x_qdd_922d4 : Constant  Value=x_qdd
  Constant_x_qdd_ba7b6 : Constant  Value=x_qdd
  Constant_x_qdd_f6de4 : Constant  Value=x_qdd
  Divide_0368d : Product  Inputs=*/
  Divide_24cf8 : Product  Inputs=*/
  Divide_3346b : Product  Inputs=*/
  Divide_5b634 : Product  Inputs=*/
  Divide_6d4be : Product  Inputs=*/
  Divide_9244e : Product  Inputs=*/
  Divide_98562 : Product  Inputs=*/
  Divide_d83e3 : Product  Inputs=*/
  Power_5799e : Math  Operator=pow
  Product_0818e : Product
  Product_0df4e : Product
  Product_1dd40 : Product
  Product_2977a : Product
  Product_33224 : Product
  Product_4925d : Product
  Product_4cdc7 : Product
  Product_67d34 : Product
  Product_8a7b2 : Product
  Product_94c27 : Product
  Product_ab116 : Product
  Product_caff9 : Product
  Product_cf49c : Product
  Product_decd9 : Product
  Product_edfa2 : Product
  Product_ef113 : Product
  Product_fcd0a : Product
  Subtract_0624a : Sum  Inputs=+-
  Subtract_2f238 : Sum  Inputs=+-
  Subtract_3c532 : Sum  Inputs=+-
  Subtract_7766b : Sum  Inputs=+-
  Subtract_a9d3f : Sum  Inputs=+-
  Subtract_b2620 : Sum  Inputs=+-
  Subtract_bcf3c : Sum  Inputs=+-
  Subtract_e8834 : Sum  Inputs=+-
  Blockout_d_psi_gq_SG_D_2_ad782 : Outport
  wires:
  Constant_x_l_0e339/1 -> Product_2977a/2
  Constant_x_l_f13c9/1 -> Product_cf49c/2
  Constant_x_qd_50550/1 -> Subtract_0624a/1
  Constant_x_l_eb83f/1 -> Product_0818e/2
  Constant_x_qdd_922d4/1 -> Subtract_e8834/2
  Constant_-1_d4ea1/1 -> Product_8a7b2/1
  Constant_-1_7bff6/1 -> Product_decd9/1
  State_psi_gq_SG_D_2_b3a61/1 -> Add_20575/1
  Constant_x_qdd_f6de4/1 -> Subtract_0624a/2
  Constant_x_qd_cf296/1 -> Subtract_e8834/1
  Constant_x_l_39996/1 -> Product_8a7b2/2
  Constant_x_l_376da/1 -> Product_decd9/2
  Product_8a7b2/1 -> Add_c92ee/1
  Product_decd9/1 -> Add_a8348/1
  Constant_x_l_e3787/1 -> Product_1dd40/2
  Constant_x_l_16659/1 -> Product_ef113/2
  Constant_x_qd_391fb/1 -> Add_c92ee/2
  Constant_x_qdd_5fede/1 -> Add_a8348/2
  Constant_-1_45f20/1 -> Product_1dd40/1
  Constant_x_qd_793df/1 -> Add_4caf7/2
  Constant_x_qdd_40652/1 -> Add_b9f45/2
  State_psi_gq_SG_D_2_c36e1/1 -> Product_4925d/1
  Add_c92ee/1 -> Divide_0368d/2
  Add_a8348/1 -> Product_4925d/2
  Constant_x_qd_e6196/1 -> Subtract_2f238/2
  Product_1dd40/1 -> Add_0193e/1
  Constant_x_qd_a0516/1 -> Add_0193e/2
  State_psi_kq_SG_D_2_ca188/1 -> Product_fcd0a/1
  Divide_9244e/1 -> Subtract_b2620/1
  Subtract_0624a/1 -> Product_fcd0a/2
  Product_4925d/1 -> Divide_9244e/1
  Add_0193e/1 -> Divide_9244e/2
  Add_0220b/1 -> Product_ab116/2
  Product_fcd0a/1 -> Divide_0368d/1
  Constant_-1_6e161/1 -> Product_ef113/1
  Divide_0368d/1 -> Subtract_b2620/2
  Constant_-1_72844/1 -> Product_2977a/1
  Constant_-1_01377/1 -> Product_cf49c/1
  Product_ef113/1 -> Add_b5b3c/1
  Constant_x_qdd_0fcfe/1 -> Subtract_a9d3f/2
  Constant_x_qd_d1c64/1 -> Add_b5b3c/2
  Subtract_b2620/1 -> Add_0220b/1
  Constant_-1_25aff/1 -> Product_0818e/1
  State_psi_q_SG_D_2_75609/1 -> Add_0220b/2
  Product_2977a/1 -> Add_4caf7/1
  Product_cf49c/1 -> Add_b9f45/1
  Constant_-1_b1935/1 -> Product_94c27/1
  Product_ab116/1 -> Divide_3346b/1
  Constant_x_l_082e8/1 -> Product_94c27/2
  Product_4cdc7/1 -> Add_b6586/2
  Constant_x_qd_ac3c1/1 -> Subtract_a9d3f/1
  Add_b5b3c/1 -> Product_ab116/1
  State_psi_gq_SG_D_2_ee37c/1 -> Product_0df4e/1
  Add_4caf7/1 -> Divide_d83e3/2
  Add_b9f45/1 -> Product_0df4e/2
  Product_94c27/1 -> Add_ccca3/1
  Constant_x_qd_9ed49/1 -> Add_ccca3/2
  State_psi_kq_SG_D_2_03d84/1 -> Product_edfa2/1
  Subtract_a9d3f/1 -> Product_edfa2/2
  Divide_d83e3/1 -> Subtract_3c532/2
  State_psi_kq_SG_D_2_80cf3/1 -> Add_20575/2
  Product_edfa2/1 -> Divide_d83e3/1
  Constant_x_qdd_ba7b6/1 -> Divide_3346b/2
  Product_0df4e/1 -> Divide_6d4be/1
  Add_ccca3/1 -> Divide_6d4be/2
  Constant_-1_e2de3/1 -> Product_caff9/1
  Subtract_e8834/1 -> Product_caff9/2
  Add_20575/1 -> Subtract_bcf3c/1
  Divide_3346b/1 -> Subtract_bcf3c/2
  Product_0818e/1 -> Add_6d4ea/1
  Constant_x_qd_e1c54/1 -> Add_6d4ea/2
  Divide_6d4be/1 -> Subtract_3c532/1
  Product_caff9/1 -> Product_67d34/1
  Subtract_bcf3c/1 -> Product_67d34/2
  Add_6d4ea/1 -> Power_5799e/1
  Constant_2.0_b84df/1 -> Power_5799e/2
  Subtract_3c532/1 -> Add_5e930/1
  State_psi_q_SG_D_2_7ca39/1 -> Add_5e930/2
  Product_67d34/1 -> Divide_5b634/1
  Power_5799e/1 -> Divide_5b634/2
  Add_5e930/1 -> Divide_98562/1
  Constant_x_qdd_44acf/1 -> Divide_98562/2
  Constant_x_q_98001/1 -> Subtract_2f238/1
  Divide_5b634/1 -> Subtract_7766b/1
  Divide_98562/1 -> Subtract_7766b/2
  Divide_24cf8/1 -> Blockout_d_psi_gq_SG_D_2_ad782/1
  Constant_-1_7bdb7/1 -> Product_33224/1
  State_psi_gq_SG_D_2_f5a80/1 -> Product_33224/2
  Subtract_2f238/1 -> Product_4cdc7/1
  Subtract_7766b/1 -> Product_4cdc7/2
  Product_33224/1 -> Add_b6586/1
  Add_b6586/1 -> Divide_24cf8/1
  Constant_T_qd_eceb8/1 -> Divide_24cf8/2

== system IEEE9_case/SG_D_2/d_psi_kq_SG_D_2_block ==
  note: d_psi_kq_SG_D_2 in IEEE9_case
      | $-\frac{\psi _{\mathrm{gq},\mathrm{SG},D,2}+\psi _{\mathrm{kq},\mathrm{SG},D,2}+\frac{\left(x_{l}-x_{\mathrm{qd}}\right)\,\left(\psi _{q,\mathrm{SG},D,2}+\frac{\psi _{\mathrm{gq},\mathrm{SG},D,2}\,\left(x_{l}-x_{\mathrm{qdd}}\right)}{x_{l}-x_{\mathrm{qd}}}+\frac{\psi _{\mathrm{kq},\mathrm{SG},D,2}\,\left(x_{\mathrm{qd}}-x_{\mathrm{qdd}}\right)}{x_{l}-x_{\mathrm{qd}}}\right)}{x_{\mathrm{qdd}}}}{T_{\mathrm{qdd}}}$
      | Automatically generated on 2025-11-01 08:48:53 .
  State_psi_gq_SG_D_2_d035b : Inport
  State_psi_kq_SG_D_2_6c00b : Inport  Port=2
  State_psi_gq_SG_D_2_ad537 : Inport  Port=3
  State_psi_kq_SG_D_2_d1d79 : Inport  Port=4
  State_psi_q_SG_D_2_cf35f : Inport  Port=5
  Add_15c47 : Sum
  Add_49a33 : Sum
  Add_73c8a : Sum
  Add_a556d : Sum
  Add_aa20e : Sum
  Add_e7047 : Sum
  Constant_-1_060c6 : Constant  Value=-1
  Constant_-1_16f2f : Constant  Value=-1
  Constant_-1_755bd : Constant  Value=-1
  Constant_-1_c43f5 : Constant  Value=-1
  Constant_-1_c9464 : Constant  Value=-1
  Constant_T_qdd_462f8 : Constant  Value=T_qdd
  Constant_x_l_02ad3 : Constant  Value=x_l
  Constant_x_l_0f01a : Constant  Value=x_l
  Constant_x_l_62702 : Constant  Value=x_l
  Constant_x_l_bcf13 : Constant  Value=x_l
  Constant_x_qd_5a099 : Constant  Value=x_qd
  Constant_x_qd_6673b : Constant  Value=x_qd
  Constant_x_qd_72e68 : Constant  Value=x_qd
  Constant_x_qd_9a9b6 : Constant  Value=x_qd
  Constant_x_qdd_5cfdd : Constant  Value=x_qdd
  Constant_x_qdd_5f037 : Constant  Value=x_qdd
  Constant_x_qdd_c2a1d : Constant  Value=x_qdd
  Divide_541a2 : Product  Inputs=*/
  Divide_7e6e0 : Product  Inputs=*/
  Divide_db59d : Product  Inputs=*/
  Divide_f2702 : Product  Inputs=*/
  Product_13970 : Product
  Product_20701 : Product
  Product_21d27 : Product
  Product_5d345 : Product
  Product_60142 : Product
  Product_7ffe3 : Product
  Product_90b7b : Product
  Product_ffeb1 : Product
  Subtract_2f301 : Sum  Inputs=+-
  Subtract_4b3e1 : Sum  Inputs=+-
  Subtract_a53a9 : Sum  Inputs=+-
  Blockout_d_psi_kq_SG_D_2_39ae4 : Outport
  wires:
  State_psi_kq_SG_D_2_6c00b/1 -> Subtract_2f301/2
  Constant_-1_060c6/1 -> Product_13970/1
  Constant_-1_755bd/1 -> Product_7ffe3/1
  Constant_x_l_62702/1 -> Product_7ffe3/2
  Constant_x_qdd_5f037/1 -> Add_e7047/2
  Constant_x_l_0f01a/1 -> Product_13970/2
  Constant_x_qd_5a099/1 -> Subtract_4b3e1/1
  Constant_T_qdd_462f8/1 -> Divide_7e6e0/2
  Constant_-1_c9464/1 -> Product_20701/1
  Product_7ffe3/1 -> Add_e7047/1
  Constant_x_qdd_5cfdd/1 -> Subtract_4b3e1/2
  Constant_x_l_02ad3/1 -> Product_20701/2
  Divide_7e6e0/1 -> Blockout_d_psi_kq_SG_D_2_39ae4/1
  State_psi_gq_SG_D_2_ad537/1 -> Product_21d27/1
  Add_e7047/1 -> Product_21d27/2
  Product_13970/1 -> Add_a556d/1
  Constant_x_qd_72e68/1 -> Add_a556d/2
  Product_ffeb1/1 -> Divide_541a2/1
  State_psi_kq_SG_D_2_d1d79/1 -> Product_90b7b/1
  Subtract_4b3e1/1 -> Product_90b7b/2
  Product_20701/1 -> Add_49a33/1
  Constant_x_qd_6673b/1 -> Add_49a33/2
  Product_90b7b/1 -> Divide_db59d/1
  Product_21d27/1 -> Divide_f2702/1
  Add_a556d/1 -> Divide_f2702/2
  Add_49a33/1 -> Divide_db59d/2
  State_psi_q_SG_D_2_cf35f/1 -> Add_aa20e/2
  Constant_-1_16f2f/1 -> Product_60142/1
  Constant_x_l_bcf13/1 -> Product_60142/2
  Divide_f2702/1 -> Subtract_a53a9/1
  Divide_db59d/1 -> Subtract_a53a9/2
  Product_60142/1 -> Add_73c8a/1
  Constant_x_qd_9a9b6/1 -> Add_73c8a/2
  Subtract_a53a9/1 -> Add_aa20e/1
  Constant_x_qdd_c2a1d/1 -> Divide_541a2/2
  Constant_-1_c43f5/1 -> Product_5d345/1
  State_psi_gq_SG_D_2_d035b/1 -> Product_5d345/2
  Add_73c8a/1 -> Product_ffeb1/1
  Add_aa20e/1 -> Product_ffeb1/2
  Product_5d345/1 -> Subtract_2f301/1
  Subtract_2f301/1 -> Add_15c47/1
  Divide_541a2/1 -> Add_15c47/2
  Add_15c47/1 -> Divide_7e6e0/1

== system IEEE9_case/SG_D_2/d_psi_q_SG_D_2_block ==
  note: d_psi_q_SG_D_2 in IEEE9_case
      | $2\,\pi \,f_{0}\,\left(v_{d,\mathrm{SG},D,2}\,\cos\left(\theta _{\mathrm{SG},D,2}\right)+v_{q,\mathrm{SG},D,2}\,\sin\left(\theta _{\mathrm{SG},D,2}\right)-\frac{R_{a}\,\left(\psi _{q,\mathrm{SG},D,2}+\frac{\psi _{\mathrm{gq},\mathrm{SG},D,2}\,\left(x_{l}-x_{\mathrm{qdd}}\right)}{x_{l}-x_{\mathrm{qd}}}+\frac{\psi _{\mathrm{kq},\mathrm{SG},D,2}\,\left(x_{\mathrm{qd}}-x_{\mathrm{qdd}}\right)}{x_{l}-x_{\mathrm{qd}}}\right)}{x_{\mathrm{qdd}}}-\frac{\psi _{d,\mathrm{SG},D,2}\,w_{\mathrm{SG},D,2}}{2\,f_{0}\,\pi }\right)$
      | Automatically generated on 2025-11-01 08:48:36 .
  State_psi_gq_SG_D_2_c07ab : Inport
  State_psi_kq_SG_D_2_3ead0 : Inport  Port=2
  State_psi_q_SG_D_2_c5dff : Inport  Port=3
  Input_v_d_SG_D_2_9bfd5 : Inport  Port=4
  State_theta_SG_D_2_4da9a : Inport  Port=5
  Input_v_q_SG_D_2_22342 : Inport  Port=6
  State_theta_SG_D_2_bef8f : Inport  Port=7
  State_psi_d_SG_D_2_94ada : Inport  Port=8
  State_w_SG_D_2_e3f21 : Inport  Port=9
  Add_02cb7 : Sum
  Add_0b507 : Sum
  Add_0d54a : Sum
  Add_4c221 : Sum
  Add_6ec66 : Sum
  Constant_-1_12a03 : Constant  Value=-1
  Constant_-1_6662c : Constant  Value=-1
  Constant_-1_89619 : Constant  Value=-1
  Constant_-2.0_09909 : Constant  Value=-2.0
  Constant_2.0_e0357 : Constant  Value=2.0
  Constant_R_a_6f0dd : Constant  Value=R_a
  Constant_f0_3330d : Constant  Value=f0
  Constant_f0_b17fd : Constant  Value=f0
  Constant_pi_b5aea : Constant  Value=pi
  Constant_pi_fe2cc : Constant  Value=pi
  Constant_x_l_9a144 : Constant  Value=x_l
  Constant_x_l_dd70a : Constant  Value=x_l
  Constant_x_l_f7bf9 : Constant  Value=x_l
  Constant_x_qd_6b600 : Constant  Value=x_qd
  Constant_x_qd_7ce86 : Constant  Value=x_qd
  Constant_x_qd_7e969 : Constant  Value=x_qd
  Constant_x_qdd_493f9 : Constant  Value=x_qdd
  Constant_x_qdd_b00f4 : Constant  Value=x_qdd
  Constant_x_qdd_d28a1 : Constant  Value=x_qdd
  Divide_0b5a1 : Product  Inputs=*/
  Divide_3e5ed : Product  Inputs=*/
  Divide_c3d5e : Product  Inputs=*/
  Divide_d5c3f : Product  Inputs=*/
  MathFunc_cos_824af : Trigonometry  Operator=cos
  MathFunc_sin_15c63 : Trigonometry
  Product_03486 : Product
  Product_1b396 : Product
  Product_375bc : Product
  Product_45a76 : Product
  Product_481a7 : Product
  Product_48f91 : Product
  Product_73474 : Product
  Product_7acda : Product
  Product_8509e : Product
  Product_9d7f4 : Product
  Product_c1f33 : Product
  Product_c4a75 : Product
  Product_d7ba2 : Product
  Product_fe332 : Product
  Subtract_0899f : Sum  Inputs=+-
  Subtract_2758a : Sum  Inputs=+-
  Subtract_2d98e : Sum  Inputs=+-
  Subtract_58e8b : Sum  Inputs=+-
  Blockout_d_psi_q_SG_D_2_d035a : Outport
  wires:
  Constant_x_qdd_d28a1/1 -> Subtract_2758a/2
  Constant_x_l_dd70a/1 -> Product_481a7/2
  Constant_-1_89619/1 -> Product_1b396/1
  Constant_x_l_f7bf9/1 -> Product_1b396/2
  Product_1b396/1 -> Add_4c221/1
  Constant_pi_fe2cc/1 -> Product_48f91/2
  State_psi_gq_SG_D_2_c07ab/1 -> Product_8509e/1
  Constant_x_l_9a144/1 -> Product_73474/2
  State_w_SG_D_2_e3f21/1 -> Product_375bc/2
  Constant_x_qd_6b600/1 -> Add_0d54a/2
  Constant_x_qdd_493f9/1 -> Add_4c221/2
  Constant_2.0_e0357/1 -> Product_48f91/1
  Constant_-1_6662c/1 -> Product_73474/1
  Constant_x_qd_7ce86/1 -> Subtract_2758a/1
  Constant_-1_12a03/1 -> Product_481a7/1
  State_psi_q_SG_D_2_c5dff/1 -> Add_0b507/2
  Add_4c221/1 -> Product_8509e/2
  Product_48f91/1 -> Product_fe332/1
  Product_73474/1 -> Add_02cb7/1
  Constant_pi_b5aea/1 -> Product_45a76/2
  Constant_f0_3330d/1 -> Product_fe332/2
  Constant_x_qd_7e969/1 -> Add_02cb7/2
  State_psi_kq_SG_D_2_3ead0/1 -> Product_03486/1
  Subtract_2758a/1 -> Product_03486/2
  Product_481a7/1 -> Add_0d54a/1
  Input_v_q_SG_D_2_22342/1 -> Product_9d7f4/1
  Product_8509e/1 -> Divide_d5c3f/1
  Product_fe332/1 -> Divide_0b5a1/2
  Add_02cb7/1 -> Divide_d5c3f/2
  Product_03486/1 -> Divide_c3d5e/1
  Add_0d54a/1 -> Divide_c3d5e/2
  Divide_d5c3f/1 -> Subtract_0899f/1
  State_theta_SG_D_2_4da9a/1 -> MathFunc_cos_824af/1
  Divide_c3d5e/1 -> Subtract_0899f/2
  Subtract_0899f/1 -> Add_0b507/1
  MathFunc_cos_824af/1 -> Product_c4a75/2
  Constant_R_a_6f0dd/1 -> Product_c1f33/1
  Add_0b507/1 -> Product_c1f33/2
  State_theta_SG_D_2_bef8f/1 -> MathFunc_sin_15c63/1
  Product_c1f33/1 -> Divide_3e5ed/1
  Product_45a76/1 -> Product_7acda/1
  Product_9d7f4/1 -> Subtract_2d98e/2
  Constant_x_qdd_b00f4/1 -> Divide_3e5ed/2
  Input_v_d_SG_D_2_9bfd5/1 -> Product_c4a75/1
  Add_6ec66/1 -> Product_d7ba2/2
  Divide_3e5ed/1 -> Subtract_58e8b/1
  Product_c4a75/1 -> Subtract_58e8b/2
  MathFunc_sin_15c63/1 -> Product_9d7f4/2
  Product_d7ba2/1 -> Blockout_d_psi_q_SG_D_2_d035a/1
  State_psi_d_SG_D_2_94ada/1 -> Product_375bc/1
  Constant_-2.0_09909/1 -> Product_45a76/1
  Product_7acda/1 -> Product_d7ba2/1
  Subtract_58e8b/1 -> Subtract_2d98e/1
  Product_375bc/1 -> Divide_0b5a1/1
  Constant_f0_b17fd/1 -> Product_7acda/2
  Subtract_2d98e/1 -> Add_6ec66/1
  Divide_0b5a1/1 -> Add_6ec66/2

== system IEEE9_case/SG_D_2/d_theta_SG_D_2_block ==
  note: d_theta_SG_D_2 in IEEE9_case
      | $w_{\mathrm{SG},D,2}-2\,\pi \,f_{0}$
      | Automatically generated on 2025-11-01 08:49:00 .
  State_w_SG_D_2_1f89c : Inport
  Add_a90cf : Sum
  Constant_-2.0_3c518 : Constant  Value=-2.0
  Constant_f0_5ddbd : Constant  Value=f0
  Constant_pi_4fd82 : Constant  Value=pi
  Product_8146e : Product
  Product_e630d : Product
  Blockout_d_theta_SG_D_2_e52e5 : Outport
  wires:
  Constant_-2.0_3c518/1 -> Product_8146e/1
  Constant_pi_4fd82/1 -> Product_8146e/2
  Add_a90cf/1 -> Blockout_d_theta_SG_D_2_e52e5/1
  Product_8146e/1 -> Product_e630d/1
  Constant_f0_5ddbd/1 -> Product_e630d/2
  Product_e630d/1 -> Add_a90cf/1
  State_w_SG_D_2_1f89c/1 -> Add_a90cf/2
